simulink model "canonBallModel4"  (R2017b)
settings: Solver=VariableStepAuto  StartTime=0.0  StopTime=30  RelTol=1e-3
libraries: simulink x1
settings Model: Creator=javed  LastModifiedBy=javed

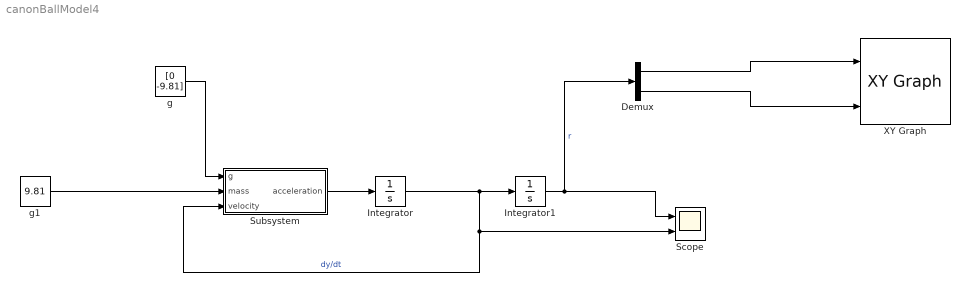
== system canonBallModel4 ==
  Demux : Demux  Outputs=2
  Integrator : Integrator  InitialCondition=[100, 100]
  Integrator1 : Integrator  InitialCondition=[0, 0]
  Scope : Scope  NumInputPorts=2
  Subsystem : Subsystem
  XY Graph : simulink/Sinks/XY Graph  xmin=0  xmax=600  ymin=-10  ymax=300  st=-1
  g : Constant  Value=[0 -9.81]
  g1 : Constant  Value=9.81
  wires:
  Integrator/1 -> Scope/2, Subsystem/3(velocity), Integrator1/1  "dy/dt"
  g/1 -> Subsystem/1(g)
  Subsystem/1("acceleration ") -> Integrator/1
  g1/1 -> Subsystem/2("mass ")
  Integrator1/1 -> Demux/1, Scope/1  "r"
  Demux/1 -> XY Graph/1
  Demux/2 -> XY Graph/2

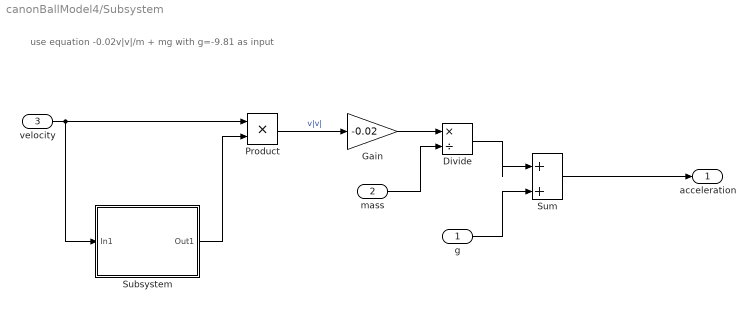
== system canonBallModel4/Subsystem ==
  note: use equation -0.02v|v|/m + mg with g=-9.81 as input
  g : Inport
  "mass " : Inport  Port=2
  velocity : Inport  Port=3
  Divide : Product  Inputs=*/
  Gain : Gain  Gain=-0.02
  Product : Product
  Subsystem : Subsystem  mask{Parameter1=0, Parameter2=0, Parameter3=0}
      mask Display: image('C:\Users\javed\Pictures\spectral.png');
  Sum : Sum  Inputs=|++
  "acceleration " : Outport
  wires:
  velocity/1 -> Subsystem/1(In1), Product/1
  Product/1 -> Gain/1  "v|v|"
  Gain/1 -> Divide/1
  "mass "/1 -> Divide/2
  Divide/1 -> Sum/1
  g/1 -> Sum/2
  Sum/1 -> "acceleration "/1
  Subsystem/1(Out1) -> Product/2

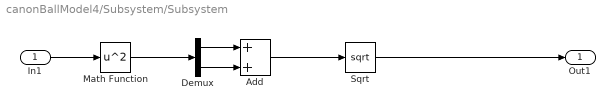
== system canonBallModel4/Subsystem/Subsystem ==
  In1 : Inport
  Add : Sum
  Demux : Demux  Outputs=2
  Math Function : Math  Operator=square  SaturateOnIntegerOverflow=on
  Sqrt : Sqrt  SaturateOnIntegerOverflow=on
  Out1 : Outport
  wires:
  In1/1 -> Math Function/1
  Math Function/1 -> Demux/1
  Demux/1 -> Add/1
  Demux/2 -> Add/2
  Add/1 -> Sqrt/1
  Sqrt/1 -> Out1/1
